simulink model "sim_emt"  (R2025a)
settings: Solver=ode23s  StartTime=0.0  StopTime=1  RelTol=1e-3
undefined symbols (not defined in the file or in its folder): bus, inf_src, line_pi, ts
libraries: sps_library x5, sps_lib x1
settings Model: SimulationMode=accelerator  Creator=sern494  LastModifiedBy=paul

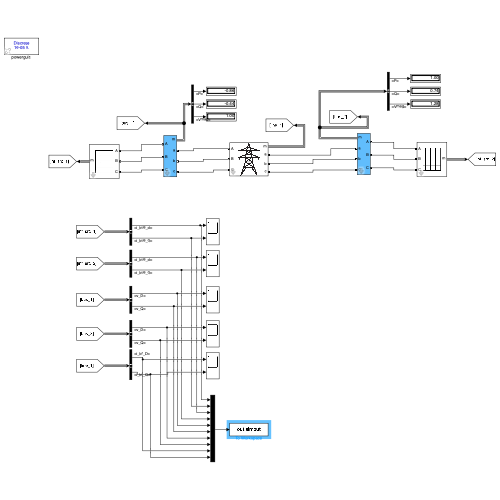
[thumbnail: Simulink's stored preview of the top-level diagram]
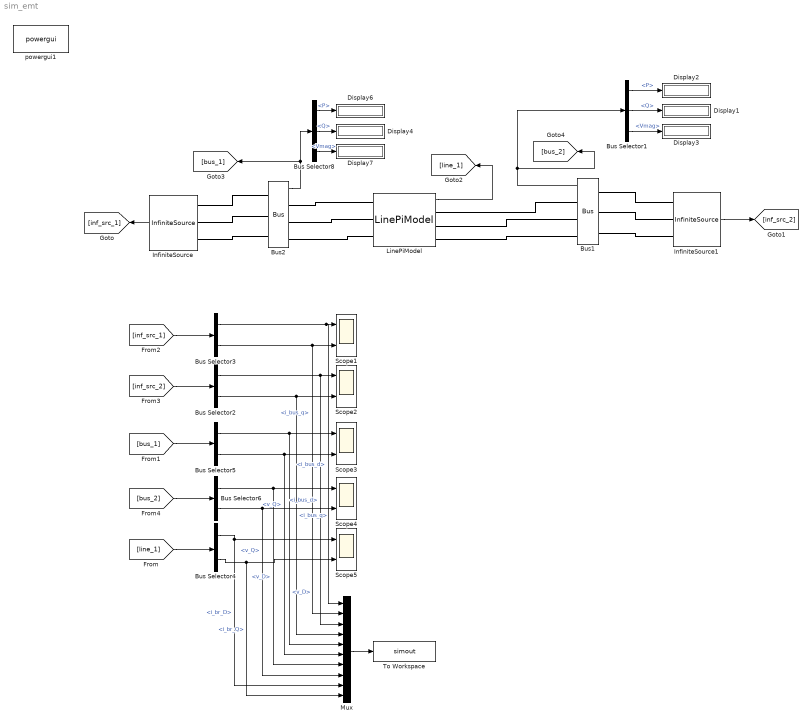
== system sim_emt ==
  Bus Selector1 : BusSelector  OutputSignals=P,Q,Vmag
  Bus Selector2 : BusSelector  OutputSignals=i_bus_d,i_bus_q
  Bus Selector3 : BusSelector  OutputSignals=i_bus_d,i_bus_q
  Bus Selector4 : BusSelector  OutputSignals=i_br_D,i_br_Q
  Bus Selector5 : BusSelector  OutputSignals=v_D,v_Q
  Bus Selector6 : BusSelector  OutputSignals=v_D,v_Q
  Bus Selector8 : BusSelector  OutputSignals=P,Q,Vmag
  Bus1 : sps_library/Bus  s=bus{2}  sbase=100000000  vbase=230000  fbase=60
  Bus2 : sps_library/Bus  s=bus{1}  sbase=100000000  vbase=230000  fbase=60
  Display{1..4,6..7} (6 alike) : Display
      settings: Format=bank
  InfiniteSource : sps_library/InfiniteSource  s=inf_src{1}
  InfiniteSource1 : sps_library/InfiniteSource  s=inf_src{2}
  LinePiModel : sps_library/LinePiModel  s=line_pi{1}
  Mux : Mux  Inputs=10
  Scope{1..5} (5 alike) : Scope  NumInputPorts=2
      Scope1 settings: ActiveDisplayYMinimum=-1  ActiveDisplayYMaximum=1  DataLoggingVariableName=ScopeData4
      Scope2 settings: ActiveDisplayYMinimum=-1  ActiveDisplayYMaximum=1
      Scope3 settings: ActiveDisplayYMinimum=-1  ActiveDisplayYMaximum=1
      Scope4 settings: ActiveDisplayYMinimum=-1  ActiveDisplayYMaximum=1  DataLoggingVariableName=ScopeData2
      Scope5 settings: ActiveDisplayYMinimum=-1  ActiveDisplayYMaximum=1  DataLoggingVariableName=ScopeData3
  To Workspace : ToWorkspace  VariableName=simout  SaveFormat=Timeseries  SampleTime=10^(-3)
  powergui1 : sps_lib/powergui  Priority=1  SimulationMode=Discrete  SampleTime=ts  frequency=60  Iterations=50  frequencyindice=60  Pbase=100e6  ErrMax=1e-4  UnitsV=kV  UnitsW=MW  buscounter=0  FunctionMessages=off  echomessages=off  EnableUseOfTLC=off  CurrentSourceSwitches=off  DisableSnubberDevices=off  DisableRonSwitches=off  DisableVfSwitches=off  DisplayEquations=off  AutomaticDiscreteSolvers=off  SolverType=Tustin/Backward Euler (TBE)  Interpol=off  ExternalGateDelay=off  methode=off  Ts=100  x0status=blocks  SPID=on  SwTol=0  HookPort=off  NonlinearTolerance=1e-4  nMaxIteration=100  ContinueOnMaxIteration=off  RestoreLinks=warning  ResistiveCurrentMeasurement=off  Frange=[0:2:500]  Ylog=off  Xlog=on  ShowGrid=off  save=off  variable=ZData  structure=0  ZoomFFT=off  StartTime=0.0  cycles=1  DisplayStyle=1  fundamental=60  FreqAxis=off  MaxFrequency=1000  frequencyindicesteady=1  RmsSteady=1  display=off
  wires:
  Bus Selector8/3 -> Display7/1  "<Vmag>"
  Bus Selector8/2 -> Display4/1  "<Q>"
  Bus Selector8/1 -> Display6/1  "<P>"
  Bus Selector1/1 -> Display2/1  "<P>"
  Bus Selector1/2 -> Display1/1  "<Q>"
  Bus Selector1/3 -> Display3/1  "<Vmag>"
  Bus Selector3/1 -> Mux/1, Scope1/1  "<i_bus_d>"
  Bus Selector3/2 -> Mux/2, Scope1/2  "<i_bus_q>"
  InfiniteSource/1 -> [inf_src_1]
  InfiniteSource1/1 -> [inf_src_2]
  [inf_src_1] -> Bus Selector3/1
  [inf_src_2] -> Bus Selector2/1
  Bus Selector2/1 -> Mux/3, Scope2/1  "<i_bus_d>"
  Bus Selector2/2 -> Mux/4, Scope2/2  "<i_bus_q>"
  LinePiModel/1 -> [line_1]
  [line_1] -> Bus Selector4/1
  [bus_1] -> Bus Selector5/1
  [bus_2] -> Bus Selector6/1
  Bus Selector5/1 -> Mux/5, Scope3/1  "<v_D>"
  Bus Selector5/2 -> Mux/6, Scope3/2  "<v_Q>"
  Bus Selector6/1 -> Mux/7, Scope4/1  "<v_D>"
  Bus Selector6/2 -> Mux/8, Scope4/2  "<v_Q>"
  Bus Selector4/2 -> Mux/10, Scope5/2  "<i_br_Q>"
  Bus Selector4/1 -> Scope5/1, Mux/9  "<i_br_D>"
  Mux/1 -> To Workspace/1
  Bus2/1 -> Bus Selector8/1, [bus_1]
  Bus1/1 -> [bus_2], Bus Selector1/1
  connections:
  InfiniteSource/LConn1 -- Bus2/LConn1
  InfiniteSource/LConn2 -- Bus2/LConn2
  InfiniteSource/LConn3 -- Bus2/LConn3
  Bus2/RConn1 -- LinePiModel/LConn1
  Bus2/RConn2 -- LinePiModel/LConn2
  Bus2/RConn3 -- LinePiModel/LConn3
  Bus1/LConn1 -- InfiniteSource1/LConn1
  Bus1/LConn2 -- InfiniteSource1/LConn2
  Bus1/LConn3 -- InfiniteSource1/LConn3
  LinePiModel/RConn1 -- Bus1/RConn1
  LinePiModel/RConn2 -- Bus1/RConn2
  LinePiModel/RConn3 -- Bus1/RConn3
